simulink model "MPCcontrol_red"  (R2015b)
settings: Solver=FixedStepAuto  StartTime=0.0  StopTime=30  FixedStep=0.01  MaxStep=0.005  RelTol=1e-3
InitFcn:
  | Ts=0.01;
  | dPL22=2*dPL2;
values from neighbouring files (symbols this model uses):
  A = [-12.5 2.5 0 0 0 0 0 0 -2.5 5.99880023995 0 0 ... (49 elements, 7x7)]    [MPCred2_out.mat]    (also in ObserverModel_2area.m = [-1/Tg1     0      -1/(R1*Tg1)   0       0       0        0)
  a = [-0.183721545007 -4.16205267369 0.0280289737335 0.00211143008158 -0.00295769226235 4.21561257449 -0.0928706956511 0.0167588644921 0.0262265264472 -0.151880268826 0.0114058405038 0.0121896199193 ... (25 elements, 5x5)]    [MPCred2_out.mat]
  B = [12.5 0 0 0 0 0 0 0 0 0 0 12.5 ... (28 elements, 7x4)]    [MPCred2_out.mat]    (also in ObserverModel_2area.m = [ 1/Tg1 0    0    0)
  b = [0.119647093263 -0.748458880856 0.451632878926 0.842051620506 -0.83548856174 -0.119204132238 0.549473893827 0.494122210734 0.80649011207 0.765264017215 1.38884507042 0.624028370982 ... (20 elements, 5x4)]    [MPCred2_out.mat]
  C = [0 0 0 0 0.425 0 1 -1 0 0 0 0 ... (14 elements, 2x7)]    [MPCred2_out.mat]    (also in ObserverModel_2area.m = [0 0 B1  1 0 0 0)
  c = [-1.3479218625  0.840223590308  1.08531793878  -0.745584512523  -0.825863541108; 1.15752440119  -0.901756501932  1.14672775481  -0.896662736397  0.793660449878]    [MPCred2_out.mat]
  dPL1 = 0    [MPCred2_out.mat]    (also in ObserverModel_2area.m = 0.1)
  dPL2 = 0.1    [MPCred2_out.mat]    (also in ObserverModel_2area.m = 0)
  Lred = [-22.0795462537  14.5599706676; -174.253205306  218.88785772; 35.2087682203  90.7537633869; 34.9986418096  82.9463604088; -189.169737333  258.207746518]    [MPCred2_out.mat]    (also in ObserverModel_2area.m = place(a',c',Pole_redobs)')
settings Model: Creator=Majidi  LastModifiedBy=Admin
settings DataIOCC: SaveFormat=Array
settings OptimizationCC: ExpressionDepthLimit=2147483647
settings DebuggingCC: UnderspecifiedInitializationDetection=Classic  MergeDetectMultiDrivingBlocksExec=none  SolverPrmCheckMsg=warning  StateNameClashWarn=warning
settings HardwareCC: ProdBitPerPointer=32  ProdLargestAtomicFloat=None  ProdIntDivRoundTo=Undefined  ProdEndianess=Unspecified  ProdWordSize=32  ProdHWDeviceType=32-bit Generic
settings GRTTargetCC: GeneratePreprocessorConditionals=Disable all
settings ConfigComp: CovModelRefEnable=Off

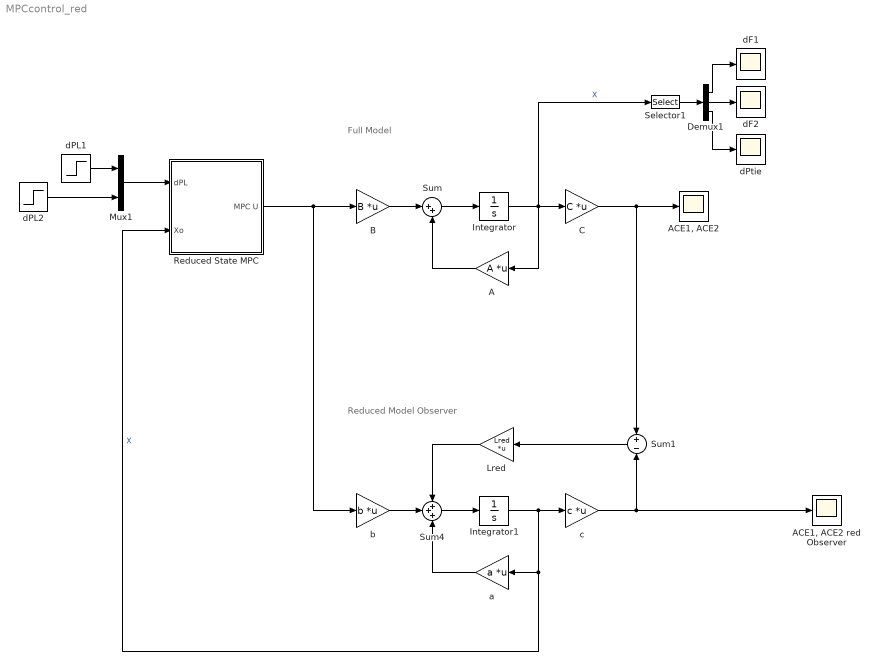
== system MPCcontrol_red ==
  note: Full Model
  note: Reduced Model Observer
  A : Gain  Gain=A  Multiplication=Matrix(K*u)
  "ACE1, ACE2" : Scope
  "ACE1, ACE2 red Observer" : Scope
  B : Gain  Gain=B  Multiplication=Matrix(K*u)
  C : Gain  Gain=C  Multiplication=Matrix(K*u)
  Demux1 : Demux  Outputs=3
  Integrator : Integrator
  Integrator1 : Integrator  InitialCondition=[0 0 0 0 0]
  Lred : Gain  Gain=Lred  Multiplication=Matrix(K*u)
  Mux1 : Mux  Inputs=2
  Reduced State MPC : Subsystem
  Selector1 : Selector  InputPortWidth=7  IndexOptions=Index vector (dialog)  Indices=[3 7 4]  OutputSizes=1
  Sum : Sum  Inputs=|++
  Sum1 : Sum  Inputs=+|-
  Sum4 : Sum  Inputs=+++
  a : Gain  Gain=a  Multiplication=Matrix(K*u)
  b : Gain  Gain=b  Multiplication=Matrix(K*u)
  c : Gain  Gain=c  Multiplication=Matrix(K*u)
  dF1 : Scope
  dF2 : Scope
  dPL1 : Step  After=dPL1  SampleTime=0
  dPL2 : Step  After=dPL22  SampleTime=0
  dPtie : Scope
  wires:
  B/1 -> Sum/1
  Sum/1 -> Integrator/1
  A/1 -> Sum/2
  Integrator/1 -> Selector1/1, A/1, C/1  "X"
  C/1 -> "ACE1, ACE2"/1, Sum1/1
  dPL1/1 -> Mux1/1
  dPL2/1 -> Mux1/2
  Mux1/1 -> Reduced State MPC/1(dPL)
  Reduced State MPC/1(MPC U) -> b/1, B/1
  b/1 -> Sum4/2
  Sum4/1 -> Integrator1/1
  a/1 -> Sum4/3
  Integrator1/1 -> c/1, Reduced State MPC/2(Xo), a/1  "X"
  c/1 -> "ACE1, ACE2 red Observer"/1, Sum1/2
  Sum1/1 -> Lred/1
  Lred/1 -> Sum4/1
  Demux1/1 -> dF1/1
  Demux1/2 -> dF2/1
  Demux1/3 -> dPtie/1
  Selector1/1 -> Demux1/1

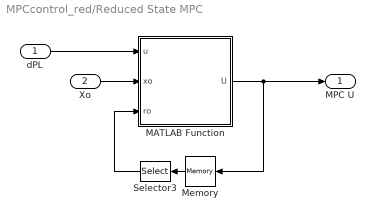
== system MPCcontrol_red/Reduced State MPC ==
  dPL : Inport
  Xo : Inport  Port=2
  MATLAB Function : MATLAB Function  TreatAsAtomicUnit=on
  Memory : Memory  X0=[0;0;0;0]
  Selector3 : Selector  InputPortWidth=4  IndexOptions=Index vector (dialog)  Indices=[1 2]  OutputSizes=1
  MPC U : Outport
  wires:
  Selector3/1 -> MATLAB Function/3(ro)
  dPL/1 -> MATLAB Function/1(u)
  MATLAB Function/1(U) -> MPC U/1, Memory/1
  Xo/1 -> MATLAB Function/2(xo)
  Memory/1 -> Selector3/1

== matlab function MPCcontrol_red/Reduced State MPC/MATLAB Function ==
  data: u input; U output; xo input; ro input
function U = MPC(u,xo,ro)

% a = [-0.420959317424693,-3.13820806605342,-0.0298204885307015,0.0576679008892296,-0.395772873014347;2.98117280324478,-0.236612704819295,0.0155819532261978,-0.0214127150611074,-0.350922004740142;-0.0614354899936130,0.0162547722166211,-0.928329453510265,2.12874683642666,0.0877635407689184;-0.0319835300890466,0.0579086425840623,-1.58486938345746,-1.05504622911219,-0.0969249879039999;-0.0894052565817334,0.341834543016131,-0.0107750027674988,-0.0298458391231411,-1.71925436254670];
% b = [0.214303509710884,-0.120905036780615,-1.30104879790810,1.00933363553808;-0.854203238784489,0.655398352882333,0.313596880325770,-0.280679849680818;0.447385035790578,0.497409488873797,-0.970960362061710,-1.04701635133746;0.814154381740479,0.830989332798914,0.0114115201092832,0.00906969204443825;0.590472996566214,-0.533322158375558,-0.0789791014161342,0.0741176806003277];
% c = [1.30268752990070,0.824146225823483,1.06448754777128,-0.801344480812097,0.540509290060342;-1.03683729871237,-0.810627753002941,1.16337573258769,-0.843475034431833,-0.593861701648441];
a=[-0.183721545006828,4.21561257448810,0.0114058405037626,0.00367408750026667,-0.236392568501128;-4.16205267369347,-0.0928706956510741,0.0121896199192519,-0.0243240089165755,0.178617279204259;0.0280289737334991,0.0167588644921035,-0.929929171517785,2.13024013261600,-0.0116349231223944;0.00211143008157946,0.0262265264472104,-1.58644954834535,-1.05975076357643,0.105825687137950;-0.00295769226235298,-0.151880268825995,0.00535290487942043,0.0829242254444511,-1.94302936634756];
b=[0.119647093263081,-0.119204132237909,1.38884507042047,-1.09514401110261;-0.748458880855902,0.549473893827396,0.624028370981700,-0.517316930291258;0.451632878925756,0.494122210734015,-0.992566756213384,-1.02935989327374;0.842051620505800,0.806490112069918,-0.00193123605376590,0.0204784281794829;-0.835488561740107,0.765264017214529,0.122997062160711,-0.114669386020992];
c=[-1.34792186249645,0.840223590308015,1.08531793877867,-0.745584512522879,-0.825863541107890;1.15752440119341,-0.901756501931565,1.14672775481068,-0.896662736396695,0.793660449878414];

yo = c*xo;  

Np = 15;h=0.01;
r = -0.25:h:0.25;
Y1 = zeros(length(r),length(r));Y2=Y1;
y=zeros(2,1);

tol = 1e-5;Ts = 0.01;
if max(abs(yo)) <= tol
    U = [ro;u];
else
    
    
for i=1:length(r)
    Pc1 = r(i);
    for j=1:length(r)
        Pc2 = r(j);
        x=xo;
        for co=1:Np
            X = x+Ts*(a*x+b*[Pc1;Pc2;u]);
            y = c*X;
            x=X;
        end
        Y1(i,j) = y(1);
        Y2(i,j) = y(2);
    end
end
err = abs(Y1)+abs(Y2);
[~,index]=min(err(:));
cul=ceil(index/length(err));
row=floor((index/length(err)-floor(index/length(err)))*length(err));
if row==0
    row=length(err);
end

U = [r(row);r(cul);u];
end
end
